simulink model "sim_sistema_3_2"  (Simulink 7.5)
settings: Solver=ode3  StartTime=0.0  StopTime=30  FixedStep=1e-4  RelTol=1e-3
values from neighbouring files (symbols this model uses):
  A = [-5 1 0;0 -2 1;0 0 -1]    [sistema_3.m]    (also in sistema_3_2.m)
  B = [0 0 1]'    [sistema_3.m]    (also in sistema_3_2.m)
settings Model: Creator=taniel.franklin  LastModifiedBy=taniel.franklin

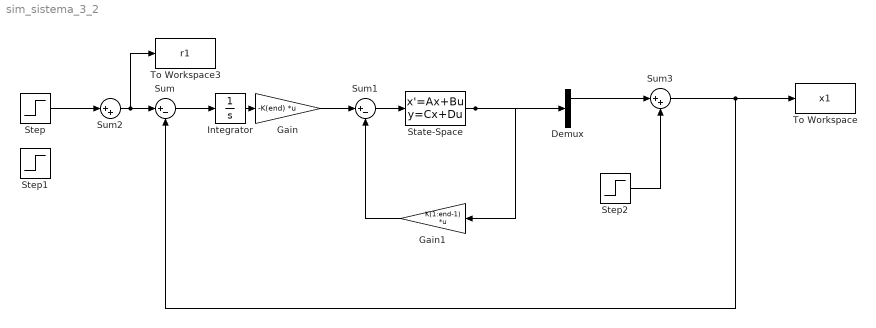
== system sim_sistema_3_2 ==
  Demux : Demux  Outputs=3
  Gain : Gain  Gain=-K(end)  Multiplication=Matrix(K*u)  ParameterDataType=fixdt(1, 16)  ParameterScaling=2^0  OutDataType=fixdt(1, 16)  OutScaling=2^0
  Gain1 : Gain  Gain=K(1:end-1)  Multiplication=Matrix(K*u)  ParameterDataType=fixdt(1, 16)  ParameterScaling=2^0  OutDataType=fixdt(1, 16)  OutScaling=2^0
  Integrator : Integrator
  State-Space : StateSpace  A=A  B=B  C=eye(3)  D=[0;0;0]
  Step : Step  Time=0.1  SampleTime=0
  Step1 : Step  Time=12  SampleTime=0
  Step2 : Step  Time=19  SampleTime=0
  Sum : Sum  Inputs=|+-  OutDataType=fixdt(1, 16)  OutScaling=2^0
  Sum1 : Sum  Inputs=|+-  OutDataType=fixdt(1, 16)  OutScaling=2^0
  Sum2 : Sum  Inputs=|++  OutDataType=fixdt(1, 16)  OutScaling=2^0
  Sum3 : Sum  Inputs=|++  OutDataType=fixdt(1, 16)  OutScaling=2^0
  To Workspace : ToWorkspace  VariableName=x1  SampleTime=-1  SaveFormat=Structure With Time
  To Workspace3 : ToWorkspace  VariableName=r1  SampleTime=-1  SaveFormat=Structure With Time
  wires:
  State-Space/1 -> Demux/1, Gain1/1
  Sum/1 -> Integrator/1
  Sum1/1 -> State-Space/1
  Step/1 -> Sum2/1
  Sum2/1 -> Sum/1, To Workspace3/1
  Gain1/1 -> Sum1/2
  Integrator/1 -> Gain/1
  Gain/1 -> Sum1/1
  Step2/1 -> Sum3/2
  Sum3/1 -> Sum/2, To Workspace/1
  Demux/1 -> Sum3/1
